simulink library "SimscapeCustomComponents_lib"  (R2025b)
settings: Solver=VariableStepAuto  StartTime=0.0  StopTime=10.0  RelTol=1e-3
undefined symbols (not defined in the file or in its folder): base, baseVdc, capacity, DiscIntNeverNeededParam, ee_sli_rtmsupport, filterInductance, freqeuncy, frequency, gcbh, gflInverter, gfmInverter, iMaxPU, Inertia, initialSOC, plantRating, solar, Ts, ups, Vac, windSystem, windTurbine
libraries: fl_lib x397, nesl_utility x171, eeGeneralControl x85, ee_lib x82, simulink x72, datacenter_lib x68, eeTransforms x38, slpidlib x24, buildingEnergy_lib x20, SimscapeFluids_lib x17, eeSinusoidalMeasurementV2 x8, eePwmGenerator x8
(part 4 of 24)

== system SimscapeCustomComponents_lib/Building Energy Management/Building/Room, Radiator, and Under-floor Piping ==
  Array Connection3 : SimscapeArrayConnection  Domain=foundation.thermal.thermal  NumScalarElements=6
  PS Selector : fl_lib/Physical Signals/Nonlinear Operators/PS Selector  ix=indxS
      settings: InternalSimscapePortConfiguration="{\"Bottom\":[],\"Left\":[{\"id\":\"I\",\"label\":\"\",\"type\":\"input\"}],\"Right\":[{\"id\":\"O\",\"label\":\"\",\"type\":\"output\"}],\"Top\":[]}"
  PS Selector1 : fl_lib/Physical Signals/Nonlinear Operators/PS Selector  ix=indxV
      settings: InternalSimscapePortConfiguration="{\"Bottom\":[],\"Left\":[{\"id\":\"I\",\"label\":\"\",\"type\":\"input\"}],\"Right\":[{\"id\":\"O\",\"label\":\"\",\"type\":\"output\"}],\"Top\":[]}"
  Room Underfloor Piping : buildingEnergy_lib/Room Underfloor Piping  pipeHydrDia=pipeHydrDiaUFP m  pipeLength=pipeLenUFP m  pipeArea=pipeCrossSectionalAreaUFP m^2  pipeRoughness=pipeRoughnessUFP m  htc=htc W/(K*m^2)  iniTemperature=iniT K
      settings: InternalSimscapePortConfiguration="{\"Bottom\":[],\"Left\":[{\"id\":\"TL_V\",\"label\":\"V\",\"type\":\"input\"},{\"id\":\"TL_A\",\"label\":\"A\",\"type\":\"foundation.thermal_liquid.thermal_liquid\"}],\"Right\":[{\"id\":\"M\",\"label\":\"R\",\"type\":\"foundation.thermal.thermal\"},{\"id\":\"TL_B\",\"label\":\"B\",\"type\":\"foundation.thermal_liquid.thermal_liquid\"}],\"Top\":[]}"
  Room Volume1 : buildingEnergy_lib/Room Volume  N1=1  N2=6  iniT=iniT K  length=roomLen m  width=roomWid m  height=roomHgt m
      settings: InternalSimscapePortConfiguration="{\"Bottom\":[],\"Left\":[{\"id\":\"S\",\"label\":\"S\",\"type\":\"input\"}],\"Right\":[{\"id\":\"T\",\"label\":\"T\",\"type\":\"output\"}],\"Top\":[{\"id\":\"M1\",\"label\":\"M1\",\"type\":\"foundation.thermal.thermal\"},{\"id\":\"M2\",\"label\":\"M2\",\"type\":\"foundation.thermal.thermal\"}]}"
  Room Wall Radiator : buildingEnergy_lib/Room Wall Radiator  pipeHydrDia=pipeHydrDiaR m  pipeLength=pipeLenR m  pipeArea=pipeCrossSectionalAreaR m^2  pipeRoughness=pipeRoughnessR m  htc=htc W/(K*m^2)  iniTemperature=iniT K
      settings: InternalSimscapePortConfiguration="{\"Bottom\":[],\"Left\":[{\"id\":\"TL_V\",\"label\":\"V\",\"type\":\"input\"},{\"id\":\"TL_A\",\"label\":\"A\",\"type\":\"foundation.thermal_liquid.thermal_liquid\"}],\"Right\":[{\"id\":\"M\",\"label\":\"R\",\"type\":\"foundation.thermal.thermal\"},{\"id\":\"TL_B\",\"label\":\"B\",\"type\":\"foundation.thermal_liquid.thermal_liquid\"}],\"Top\":[]}"
  Thermal Resistance : fl_lib/Thermal/Thermal Elements/Thermal Resistance  resistance=thermalResFloor K/W  T_specify=off  T_priority=None  T=0 K  T_nominal_specify=off  T_nominal_value=1  T_nominal_unit=K  Q_specify=off  Q_priority=None  Q=0 W  Q_nominal_specify=off  Q_nominal_value=1  Q_nominal_unit=W
  ar1 : fl_lib/Thermal/Thermal Elements/Convective Heat Transfer  thermal_type=foundation.enum.constant_variable.constant  area=roomLen*roomWid m^2  heat_tr_coeff=htc W/(K*m^2)  min_heat_tr_coeff=1e-3 W/(K*m^2)  T_specify=off  T_priority=None  T=0 K  T_nominal_specify=off  T_nominal_value=1  T_nominal_unit=K  Q_specify=off  Q_priority=None  Q=0 W  Q_nominal_specify=off  Q_nominal_value=1  Q_nominal_unit=W
  ar3 : fl_lib/Thermal/Thermal Elements/Convective Heat Transfer  thermal_type=foundation.enum.constant_variable.constant  area=roomHgt*roomWid m^2  heat_tr_coeff=htc W/(K*m^2)  min_heat_tr_coeff=1e-3 W/(K*m^2)  T_specify=off  T_priority=None  T=0 K  T_nominal_specify=off  T_nominal_value=1  T_nominal_unit=K  Q_specify=off  Q_priority=None  Q=0 W  Q_nominal_specify=off  Q_nominal_value=1  Q_nominal_unit=W
  ar4 : fl_lib/Thermal/Thermal Elements/Convective Heat Transfer  thermal_type=foundation.enum.constant_variable.constant  area=roomLen*roomHgt m^2  heat_tr_coeff=htc W/(K*m^2)  min_heat_tr_coeff=1e-3 W/(K*m^2)  T_specify=off  T_priority=None  T=0 K  T_nominal_specify=off  T_nominal_value=1  T_nominal_unit=K  Q_specify=off  Q_priority=None  Q=0 W  Q_nominal_specify=off  Q_nominal_value=1  Q_nominal_unit=W
  ar5 : fl_lib/Thermal/Thermal Elements/Convective Heat Transfer  thermal_type=foundation.enum.constant_variable.constant  area=roomHgt*roomWid m^2  heat_tr_coeff=htc W/(K*m^2)  min_heat_tr_coeff=1e-3 W/(K*m^2)  T_specify=off  T_priority=None  T=0 K  T_nominal_specify=off  T_nominal_value=1  T_nominal_unit=K  Q_specify=off  Q_priority=None  Q=0 W  Q_nominal_specify=off  Q_nominal_value=1  Q_nominal_unit=W
  ar6 : fl_lib/Thermal/Thermal Elements/Convective Heat Transfer  thermal_type=foundation.enum.constant_variable.constant  area=roomLen*roomHgt m^2  heat_tr_coeff=htc W/(K*m^2)  min_heat_tr_coeff=1e-3 W/(K*m^2)  T_specify=off  T_priority=None  T=0 K  T_nominal_specify=off  T_nominal_value=1  T_nominal_unit=K  Q_specify=off  Q_priority=None  Q=0 W  Q_nominal_specify=off  Q_nominal_value=1  Q_nominal_unit=W
  ar7 : fl_lib/Thermal/Thermal Elements/Convective Heat Transfer  thermal_type=foundation.enum.constant_variable.constant  area=pipeLenR*pipeHydrDiaR m^2  heat_tr_coeff=htc W/(K*m^2)  min_heat_tr_coeff=1e-3 W/(K*m^2)  T_specify=off  T_priority=None  T=0 K  T_nominal_specify=off  T_nominal_value=1  T_nominal_unit=K  Q_specify=off  Q_priority=None  Q=0 W  Q_nominal_specify=off  Q_nominal_value=1  Q_nominal_unit=W
  ar8 : fl_lib/Thermal/Thermal Elements/Convective Heat Transfer  thermal_type=foundation.enum.constant_variable.constant  area=pipeLenUFP*pipeHydrDiaUFP/2 m^2  heat_tr_coeff=htc W/(K*m^2)  min_heat_tr_coeff=1e-3 W/(K*m^2)  T_specify=off  T_priority=None  T=0 K  T_nominal_specify=off  T_nominal_value=1  T_nominal_unit=K  Q_specify=off  Q_priority=None  Q=0 W  Q_nominal_specify=off  Q_nominal_value=1  Q_nominal_unit=W
  V : PMIOPort  Side=Left
  S : PMIOPort  Port=2  Side=Left
  W4 : PMIOPort  Port=3  Side=Left
  TL_A : PMIOPort  Port=4  Side=Left
  W3 : PMIOPort  Port=5  Side=Left
  TL_B : PMIOPort  Port=6  Side=Right
  W2 : PMIOPort  Port=7  Side=Right
  T : PMIOPort  Port=8  Side=Right
  W1 : PMIOPort  Port=9  Side=Right
  Bottom : PMIOPort  Port=10  Side=Right
  Top : PMIOPort  Port=11  Side=Left
  connections:
  TL_B/RConn1 -- Room Underfloor Piping/RConn2 -- Room Wall Radiator/RConn2
  Room Volume1/RConn1 -- T/RConn1
  TL_A/RConn1 -- Room Underfloor Piping/LConn2 -- Room Wall Radiator/LConn2
  ar6/RConn1 -- W1/RConn1
  ar5/RConn1 -- W2/RConn1
  ar4/RConn1 -- W3/RConn1
  ar3/RConn1 -- W4/RConn1
  Thermal Resistance/LConn1 -- Room Underfloor Piping/RConn1 -- ar8/LConn1
  ar7/RConn1 -- Array Connection3/LConn2
  Top/RConn1 -- ar1/RConn1
  Thermal Resistance/RConn1 -- Bottom/RConn1
  Array Connection3/LConn3 -- ar3/LConn1
  Array Connection3/LConn4 -- ar4/LConn1
  Array Connection3/LConn5 -- ar5/LConn1
  Array Connection3/LConn6 -- ar6/LConn1
  Room Wall Radiator/RConn1 -- ar7/LConn1
  ar8/RConn1 -- Array Connection3/LConn1
  V/RConn1 -- PS Selector1/LConn1
  PS Selector1/RConn1 -- Room Underfloor Piping/LConn1 -- Room Wall Radiator/LConn1
  Room Volume1/LConn1 -- PS Selector/RConn1
  PS Selector/LConn1 -- S/RConn1
  Room Volume1/LConn3 -- Array Connection3/RConn1
  ar1/LConn1 -- Room Volume1/LConn2

== system SimscapeCustomComponents_lib/Building Energy Management/HVAC/Air Water Heat Pump (TL) ==
  ActualFlowrate : fl_lib/Physical Signals/Nonlinear Operators/PS Max  ZeroCross=true
      settings: InternalSimscapePortConfiguration="{\"Bottom\":[],\"Left\":[{\"id\":\"I1\",\"label\":\"\",\"type\":\"input\"},{\"id\":\"I2\",\"label\":\"\",\"type\":\"input\"}],\"Right\":[{\"id\":\"O\",\"label\":\"\",\"type\":\"output\"}],\"Top\":[]}"
  Air Water Heat Pump : buildingEnergy_lib/Air Water Heat Pump  nominalCapacityA=heatingCapacityA kW  seasonalCOPvalA=heatingCoPA  nominalCapacityB=heatingCapacityB kW  seasonalCOPvalB=heatingCoPB  nominalCapacityC=heatingCapacityC kW  seasonalCOPvalC=heatingCoPC  nominalCapacityD=heatingCapacityD kW  seasonalCOPvalD=heatingCoPD  nominalCapacityE=coolingCapacityE kW  seasonalCOPvalE=coolingCoPE  nominalCapacityF=coolingCapacityF kW  seasonalCOPvalF=coolingCoPF  backupElecHeater=elecHeaterPower kW  wInletOpRangeUpp=waterOpTempMax K  wInletOpRangeLow=waterOpTempMin K  airTemperatureVector=273 + [-2, -2, 7, 7, 35, 35]  waterTemperatureVector=273 + [55, 65, 35, 45, 18, 7]  waterSpHeat=4186 J/(K*kg)  smallPower=1e-3 W  maxCOP_specify=off  maxCOP_priority=None  maxCOP=8  maxCOP_nominal_specify=off  maxCOP_nominal_value=1  maxCOP_nominal_unit=1
      settings: InternalSimscapePortConfiguration="{\"Bottom\":[{\"id\":\"Ta\",\"label\":\"Ta\",\"type\":\"input\"},{\"id\":\"Tw\",\"label\":\"Tw\",\"type\":\"input\"}],\"Left\":[{\"id\":\"Tl\",\"label\":\"Tl\",\"type\":\"input\"},{\"id\":\"Fw\",\"label\":\"Fw\",\"type\":\"input\"},{\"id\":\"Op\",\"label\":\"Op\",\"type\":\"input\"},{\"id\":\"Ep\",\"label\":\"Ep\",\"type\":\"input\"},{\"id\":\"Nd\",\"label\":\"Nd\",\"type\":\"input\"}],\"Right\":[{\"id\":\"calcCap\",\"label\":\"Q\",\"type\":\"output\"},{\"id\":\"calcCOP\",\"label\":\"COP\",\"type\":\"output\"},{\"id\":\"ePower\",\"label\":\"ePow\",\"type\":\"output\"}],\"Top\":[]}"
  Heat : fl_lib/Thermal/Thermal Sources/Controlled Heat Flow Rate Source
  InMeasDelay : fl_lib/Physical Signals/Linear Operators/PS Transfer Function  transfer_function_type=foundation.enum.transfer_function_type.lag  T=measTimelagWater s  T1=2 s  T2=1 s  reset_method=foundation.enum.IntegratorResetSpec.None  initial_condition_spec=foundation.enum.IntegratorICSpec.Internal  y0=initialT K
      settings: InternalSimscapePortConfiguration="{\"Bottom\":[],\"Left\":[{\"id\":\"U\",\"label\":\"\",\"type\":\"input\"}],\"Right\":[{\"id\":\"Y\",\"label\":\"\",\"type\":\"output\"}],\"Top\":[]}"
  InsTank : fl_lib/Thermal/Thermal Elements/Perfect Insulator  T_specify=off  T_priority=None  T=293.15 K  T_nominal_specify=off  T_nominal_value=1  T_nominal_unit=K
  InternalCoils : fl_lib/Thermal Liquid/Elements/Pipe (TL)  length=coilLen m  area=coilArea m^2  Dh=coilDia m  length_add=0 m  roughness=15e-6 m  Re_lam=2000  Re_tur=4000  shape_factor=64  Nu_lam=3.66  dynamic_compressibility=true  inertia=false  p0=initialP MPa  T0=initialT K  mdot0=0 kg/s  p_nominal=0.101325 MPa  T_nominal=293.15 K
  MinFlowValue : fl_lib/Physical Signals/Sources/PS Constant  constant=minWaterFlowRate kg/s
  NoDeviation : fl_lib/Physical Signals/Sources/PS Constant  constant=1
  NomDevLim : fl_lib/Physical Signals/Nonlinear Operators/PS Max  ZeroCross=true
      settings: InternalSimscapePortConfiguration="{\"Bottom\":[],\"Left\":[{\"id\":\"I1\",\"label\":\"\",\"type\":\"input\"},{\"id\":\"I2\",\"label\":\"\",\"type\":\"input\"}],\"Right\":[{\"id\":\"O\",\"label\":\"\",\"type\":\"output\"}],\"Top\":[]}"
  OutMeasDelay : fl_lib/Physical Signals/Linear Operators/PS Transfer Function  transfer_function_type=foundation.enum.transfer_function_type.lag  T=measTimelagWater s  T1=2 s  T2=1 s  reset_method=foundation.enum.IntegratorResetSpec.None  initial_condition_spec=foundation.enum.IntegratorICSpec.Internal  y0=initialT K
      settings: InternalSimscapePortConfiguration="{\"Bottom\":[],\"Left\":[{\"id\":\"U\",\"label\":\"\",\"type\":\"input\"}],\"Right\":[{\"id\":\"Y\",\"label\":\"\",\"type\":\"output\"}],\"Top\":[]}"
  Tank : SimscapeFluids_lib/Thermal Liquid/Tanks & Accumulators/Gas-Charged Accumulator (TL)  capacity=tankVolume m^3  dead_volume=4e-5 m^3  p_precharge_gauge=0 MPa  k_sh=1.4  area=0.01 m^2  stiff_coeff=1e4 MPa/m^3  damping_coeff=1e4 MPa*s/m^6  liquid_volume_specify=off  liquid_volume_priority=High  liquid_volume=5e-3 m^3  liquid_volume_nominal_specify=off  liquid_volume_nominal_value=1  liquid_volume_nominal_unit=m^3  liquid_mass_specify=off  liquid_mass_priority=None  liquid_mass=5 kg  liquid_mass_nominal_specify=off  liquid_mass_nominal_value=1  liquid_mass_nominal_unit=kg  p_I_specify=off  p_I_priority=None  p_I=0.101325 MPa  p_I_nominal_specify=off  p_I_nominal_value=1  p_I_nominal_unit=MPa  T_I_specify=on  T_I_priority=High  T_I=initialT K  T_I_nominal_specify=off  T_I_nominal_value=1  T_I_nominal_unit=K
      settings: InternalSimscapePortConfiguration="{\"Bottom\":[],\"Left\":[],\"Right\":[{\"id\":\"A\",\"label\":\"A\",\"type\":\"foundation.thermal_liquid.thermal_liquid\"},{\"id\":\"H\",\"label\":\"H\",\"type\":\"foundation.thermal.thermal\"}],\"Top\":[]}"
  Tref : fl_lib/Thermal/Thermal Elements/Thermal Reference
  TwInet : fl_lib/Thermal Liquid/Sensors/Pressure & Temperature Sensor (TL)  reference=foundation.enum.MeasurementReference.absolute  pressure=false  pressure_spec=foundation.enum.PressureMeasementSpec.Absolute  temperature=true
      settings: InternalSimscapePortConfiguration="{\"Bottom\":[{\"id\":\"T\",\"label\":\"T\",\"type\":\"output\"}],\"Left\":[{\"id\":\"A\",\"label\":\"A\",\"type\":\"foundation.thermal_liquid.thermal_liquid\"}],\"Right\":[],\"Top\":[]}"
  TwOut : fl_lib/Thermal Liquid/Sensors/Pressure & Temperature Sensor (TL)  reference=foundation.enum.MeasurementReference.absolute  pressure=false  pressure_spec=foundation.enum.PressureMeasementSpec.Absolute  temperature=true
      settings: InternalSimscapePortConfiguration="{\"Bottom\":[{\"id\":\"T\",\"label\":\"T\",\"type\":\"output\"}],\"Left\":[{\"id\":\"A\",\"label\":\"A\",\"type\":\"foundation.thermal_liquid.thermal_liquid\"}],\"Right\":[],\"Top\":[]}"
  WaterFlowRate : fl_lib/Thermal Liquid/Sources/Flow Rate Source (TL)  source_type=foundation.enum.constant_controlled.controlled  flow_type=foundation.enum.mass_volumetric_flow.mass  mass_flow=0 kg/s  volumetric_flow=0 m^3/s  power_spec=foundation.enum.power_spec.none  area=coilArea m^2
  Fw : PMIOPort  Side=Left
  Ta : PMIOPort  Port=2  Side=Left
  Op : PMIOPort  Port=3  Side=Left
  Ep : PMIOPort  Port=4  Side=Left
  Nd : PMIOPort  Port=5  Side=Left
  A : PMIOPort  Port=6  Side=Right
  B : PMIOPort  Port=7  Side=Right
  ePow : PMIOPort  Port=8  Side=Right
  COP : PMIOPort  Port=9  Side=Right
  connections:
  TwOut/LConn1 -- B/RConn1 -- InternalCoils/RConn1
  InternalCoils/LConn1 -- WaterFlowRate/RConn1 -- TwInet/LConn1
  Fw/RConn1 -- Air Water Heat Pump/LConn2 -- ActualFlowrate/LConn1
  WaterFlowRate/LConn1 -- A/RConn1 -- Tank/RConn1
  Air Water Heat Pump/LConn1 -- InMeasDelay/RConn1
  Air Water Heat Pump/LConn3 -- Op/RConn1
  InMeasDelay/LConn1 -- TwInet/RConn1
  InternalCoils/LConn2 -- Heat/RConn2
  ePow/RConn1 -- Air Water Heat Pump/RConn3
  InsTank/LConn1 -- Tank/RConn2
  NoDeviation/RConn1 -- NomDevLim/LConn2
  Air Water Heat Pump/LConn4 -- Ep/RConn1
  Air Water Heat Pump/RConn2 -- COP/RConn1
  ActualFlowrate/RConn1 -- WaterFlowRate/LConn2
  MinFlowValue/RConn1 -- ActualFlowrate/LConn2
  Air Water Heat Pump/RConn5 -- OutMeasDelay/RConn1
  Tref/LConn1 -- Heat/LConn1
  Air Water Heat Pump/LConn5 -- NomDevLim/RConn1
  TwOut/RConn1 -- OutMeasDelay/LConn1
  Nd/RConn1 -- NomDevLim/LConn1
  Air Water Heat Pump/RConn4 -- Ta/RConn1
  Heat/RConn1 -- Air Water Heat Pump/RConn1

== system SimscapeCustomComponents_lib/Building Energy Management/HVAC/Heat Source Control ==
  HeatPumpCapacity : fl_lib/Physical Signals/Sources/PS Constant  constant=capacity J/s
  MeasurementDelay : fl_lib/Physical Signals/Linear Operators/PS Transfer Function  transfer_function_type=foundation.enum.transfer_function_type.lag  T=tau s  T1=2 s  T2=1 s  reset_method=foundation.enum.IntegratorResetSpec.None  initial_condition_spec=foundation.enum.IntegratorICSpec.Internal  y0=iniT K
      settings: InternalSimscapePortConfiguration="{\"Bottom\":[],\"Left\":[{\"id\":\"U\",\"label\":\"\",\"type\":\"input\"}],\"Right\":[{\"id\":\"Y\",\"label\":\"\",\"type\":\"output\"}],\"Top\":[]}"
  NumHeatPump : fl_lib/Physical Signals/Functions/PS Gain  gain=num
  PS Divide : fl_lib/Physical Signals/Functions/PS Divide
  PS Product : fl_lib/Physical Signals/Functions/PS Product
  PS Subtract : fl_lib/Physical Signals/Functions/PS Subtract
  PS Sum of Elements : fl_lib/Physical Signals/Functions/PS Sum of Elements  sumAll=true
      settings: InternalSimscapePortConfiguration="{\"Bottom\":[],\"Left\":[{\"id\":\"I\",\"label\":\"\",\"type\":\"input\"}],\"Right\":[{\"id\":\"O\",\"label\":\"\",\"type\":\"output\"}],\"Top\":[]}"
  PS Sum of Elements2 : fl_lib/Physical Signals/Functions/PS Sum of Elements  sumAll=true
      settings: InternalSimscapePortConfiguration="{\"Bottom\":[],\"Left\":[{\"id\":\"I\",\"label\":\"\",\"type\":\"input\"}],\"Right\":[{\"id\":\"O\",\"label\":\"\",\"type\":\"output\"}],\"Top\":[]}"
  Values<0 : fl_lib/Physical Signals/Nonlinear Operators/PS Saturation  upper_limit=0 J/s  lower_limit=-inf J/s  ZeroCross=true
  Values>0 : fl_lib/Physical Signals/Nonlinear Operators/PS Saturation  upper_limit=inf J/s  lower_limit=0 J/s  ZeroCross=true
  WaterTchange : fl_lib/Physical Signals/Sources/PS Constant  constant=delT K
  Cooling : PMIOPort  Side=Left
  Heating : PMIOPort  Port=2  Side=Left
  S : PMIOPort  Port=3  Side=Left
  Ts : PMIOPort  Port=4  Side=Right
  Tr : PMIOPort  Port=5  Side=Right
  connections:
  PS Subtract/RConn1 -- PS Product/LConn1
  Tr/RConn1 -- MeasurementDelay/LConn1
  PS Subtract/LConn1 -- Ts/RConn1
  Heating/RConn1 -- PS Sum of Elements/RConn1
  Cooling/RConn1 -- PS Sum of Elements2/RConn1
  PS Sum of Elements/LConn1 -- Values>0/RConn1
  PS Sum of Elements2/LConn1 -- Values<0/RConn1
  MeasurementDelay/RConn1 -- PS Subtract/LConn2
  HeatPumpCapacity/RConn1 -- PS Divide/LConn1
  WaterTchange/RConn1 -- PS Divide/LConn2
  NumHeatPump/LConn1 -- PS Divide/RConn1
  NumHeatPump/RConn1 -- PS Product/LConn2
  S/RConn1 -- Values<0/LConn1 -- Values>0/LConn1 -- PS Product/RConn1

== system SimscapeCustomComponents_lib/Datacenter/Assemblies/Air Cooled PDU Assembly ==
  One : fl_lib/Physical Signals/Sources/PS Constant  constant=1
  PDU Racks : Subsystem  mask{nTrays=nTrays, nRacks=nRacks, trayMass=trayMass, trayCp=trayCp, trayThermalR=trayThermalR, nGPU=nGPU, gpuTDPperDie=gpuTDPperDie, gpuIdlePower=gpuIdlePower, gpuHBMpower=gpuHBMpower, gpuExponent=gpuExponent, gpuHBMutil=gpuHBMutil, gpuLeakage=gpuLeakage, gpuNominalDieT=gpuNominalDieT, gpuDieThermalC=gpuDieThermalC, gpuHeatSinkR=gpuHeatSinkR, gpuSurfArea=gpuSurfArea, gpuAmbientR=gpuAmbientR, nCPU=nCPU, cpuTDPperSocket=cpuTDPperSocket, cpuIdlePower=cpuIdlePower, cpuExponent=cpuExponent, cpuLeakage=cpuLeakage, cpuNominalDieT=cpuNominalDieT, cpuDieThermalC=cpuDieThermalC, cpuHeatSinkR=cpuHeatSinkR, cpuSurfArea=cpuSurfArea, cpuAmbientR=cpuAmbientR, initialT=initialT, htc=htc}
      mask prompts: nTrays "Number of IT trays per rack (-)"; nRacks "Number of racks (-)"; trayMass "Tray mass (kg)"; trayCp "Tray specific heat capacity (J/kg*K)"; trayThermalR "Tray to external thermal resistance (K/W)"; nGPU "Number of GPU per tray (-)"; gpuTDPperDie "GPU TDP per die (W)"; gpuIdlePower "GPU idle power (W)"; gpuHBMpower "HBM power per GPU (W)"; gpuExponent "GPU power utilization exponent (-)"; gpuHBMutil "HBM utilization as fraction of compute utilization (-)"; gpuLeakage "Leakage increase per K above nominal temperature (W/K)"; gpuNominalDieT "Nominal die temperature at TDP (K)"; gpuDieThermalC "GPU die thermal capacitance (J/K)"; gpuHeatSinkR "GPU die-heat-sink thermal resistance (K/W)"; gpuSurfArea "Surface area per die for ambient heat transfer (m^2)"; gpuAmbientR "GPU die-ambient thermal resistance (K/W)"; nCPU "Number of CPU per tray (-)"; cpuTDPperSocket "CPU TDP per socket (W)"; cpuIdlePower "CPU idle power per socket (W)"; cpuExponent "CPU power utilization exponent (-)"; cpuLeakage "Leakage increase per K above nominal temperature (W/K)"; cpuNominalDieT "Nominal die temperature at TDP (K)"; cpuDieThermalC "CPU die thermal capacitance (J/K)"; cpuHeatSinkR "CPU die-heat-sink thermal resistance (K/W)"; cpuSurfArea "Surface area per die for ambient heat transfer (m^2)"; cpuAmbientR "CPU die-ambient thermal resistance (K/W)"; initialT "Initial temperature (K)"; htc "Heat transfer coefficient to ambient (W/m^2.K)"
      settings: CopyFcn=set_param(gcbh,'LinkStatus','none');  PortSchema="{\"entries\":[{\"content\":{\"sides\":[{\"content\":{\"connectorIds\":[\"LConn1\",\"LConn2\",\"LConn3\"]},\"type\":\"ConnectorPlacement.EquallySpacedRectSide\",\"uuid\":\"1a9a884a-dab1-4495-bf62-c6b2de6c1039\"},{\"content\":{\"connectorIds\":[\"RConn1\",\"RConn2\",\"RConn3\"],\"side\":\"RIGHT\"},\"type\":\"ConnectorPlacement.EquallySpacedRectSide\",\"uuid\":\"05c53434-51c1-4fee-b885-c321dcda8b6b\"},{\"content\":{\"side\":\"TOP\"},\"type\":\"ConnectorPlacement.EquallySpacedRectSide\",\"uuid\":\"c7b5c534-d596-4858-a133-27f005e6c9d4\"},{\"content\":{\"connectorIds\":[\"RConn4\"],\"side\":\"BOTTOM\"},\"type\":\"ConnectorPlacement.EquallySpacedRectSide\",\"uuid\":\"693f3c99-4296-4d86-bfcc-da753d3e576f\"}]},\"type\":\"ConnectorPlacement.EquallySpacedConnector\",\"uuid\":\"ed91c467-c4d0-403f-af16-bac0257594fd\"}],\"packageUris\":[\"http://schema.mathworks.com/mf0/Connector/R2020b\"],\"version\":\"1.0\"}"
      mask Help: web("DocumentationPDURacks.html")
      mask DialogControl Container10 Prompt: PDU Racks
      mask DialogControl getRatingButton Prompt: Get Rating
      mask DialogControl Container9 Prompt: IT Tray
      mask DialogControl Container6 Prompt: GPU
      mask DialogControl Container7 Prompt: CPU
      mask DialogControl Container8 Prompt: Initial Conditions
      mask Display: image('icon_PDURacks.png');
  PS Product1 : fl_lib/Physical Signals/Functions/PS Product
  PS Product2 : fl_lib/Physical Signals/Functions/PS Product
  Rack Air Cooling : Subsystem  mask{nFans=nFans, flowVec=flowVec, prDropVec=prDropVec, fanEffVec=fanEffVec, fluidDen=1.28, fluidCp=1005}
      mask prompts: nFans "Number of fans (-)"; flowVec "Fan flow rate vector (m^3/s)"; prDropVec "Pressure drop vector (Pa)"; fanEffVec "Fan efficiency vector (-)"; fluidDen "Fluid density (kg/m^3)"; fluidCp "Fluid heat capacity (J/(Kg*K))"
      settings: CopyFcn=set_param(gcbh,'LinkStatus','none');
      mask Help: web("DocumentationRackAirCooling.html")
      mask DialogControl Container3 Prompt: Fans
      mask DialogControl Container4 Prompt: Fluid Properties
      mask Display: image('icon_PDUfanCooling.png');
  Thermal Multiplier : datacenter_lib/Thermal Multiplier
      settings: InternalSimscapePortConfiguration="{\"Bottom\":[],\"Left\":[{\"id\":\"A\",\"label\":\"A\",\"type\":\"foundation.thermal.thermal\"}],\"Right\":[{\"id\":\"B\",\"label\":\"B\",\"type\":\"foundation.thermal.thermal\"}],\"Top\":[{\"id\":\"Na\",\"label\":\"Na\",\"type\":\"input\"},{\"id\":\"Nb\",\"label\":\"Nb\",\"type\":\"input\"}]}"
  Thermal Multiplier1 : datacenter_lib/Thermal Multiplier
      settings: InternalSimscapePortConfiguration="{\"Bottom\":[],\"Left\":[{\"id\":\"A\",\"label\":\"A\",\"type\":\"foundation.thermal.thermal\"}],\"Right\":[{\"id\":\"B\",\"label\":\"B\",\"type\":\"foundation.thermal.thermal\"}],\"Top\":[{\"id\":\"Na\",\"label\":\"Na\",\"type\":\"input\"},{\"id\":\"Nb\",\"label\":\"Nb\",\"type\":\"input\"}]}"
  nAssemblies : fl_lib/Physical Signals/Sources/PS Constant  constant=nAssembly
  U_gpu : PMIOPort  Side=Left
  U_cpu : PMIOPort  Port=2  Side=Left
  S_fan : PMIOPort  Port=3  Side=Left
  T_gpu : PMIOPort  Port=4  Side=Right
  T_cpu : PMIOPort  Port=5  Side=Right
  P_pdu : PMIOPort  Port=6  Side=Right
  P_fan : PMIOPort  Port=7  Side=Right
  C : PMIOPort  Port=8  Side=Left
  H : PMIOPort  Port=9  Side=Right
  connections:
  Rack Air Cooling/RConn1 -- PDU Racks/RConn4
  PDU Racks/RConn3 -- T_cpu/RConn1
  PDU Racks/LConn2 -- U_cpu/RConn1
  PDU Racks/RConn2 -- T_gpu/RConn1
  Rack Air Cooling/LConn2 -- S_fan/RConn1
  PDU Racks/LConn1 -- U_gpu/RConn1
  Thermal Multiplier/RConn1 -- PDU Racks/LConn3
  nAssemblies/RConn1 -- Thermal Multiplier1/LConn3 -- PS Product1/LConn1 -- PS Product2/LConn1 -- Thermal Multiplier/LConn3
  One/RConn1 -- Thermal Multiplier1/LConn2 -- Thermal Multiplier/LConn2
  P_pdu/RConn1 -- PS Product1/RConn1
  PS Product1/LConn2 -- PDU Racks/RConn1
  PS Product2/RConn1 -- P_fan/RConn1
  PS Product2/LConn2 -- Rack Air Cooling/RConn2
  Thermal Multiplier1/RConn1 -- Rack Air Cooling/LConn1
  H/RConn1 -- Thermal Multiplier/LConn1
  C/RConn1 -- Thermal Multiplier1/LConn1

== system SimscapeCustomComponents_lib/Datacenter/Assemblies/PDU + CDU Assembly (LUT) ==
  CDU (LUT) : Subsystem  mask{numPump=numPump, flowrate_vec=flowrate_vec, capacity_vec=capacity_vec, effPump_vec=effPump_vec, prDrop_mat=prDrop_mat, speed=speed}
      mask prompts: numPump "Total number of pumps (-)"; flowrate_vec "Coolant volumetric flowrate vector (m^3/s)"; capacity_vec "Heat exchanger capacity vector (W)"; effPump_vec "Pump efficiency vector, 0-1 (-)"; prDrop_mat "Pressure drop (Pa)"; speed "Pump speed scaling (-)"
      settings: CopyFcn=set_param(gcbh,'LinkStatus','none');  PortSchema="{\"entries\":[{\"content\":{\"sides\":[{\"content\":{\"connectorIds\":[\"LConn1\",\"LConn2\"]},\"type\":\"ConnectorPlacement.EquallySpacedRectSide\",\"uuid\":\"dd9276e8-a048-49df-a05c-f18b45aafce3\"},{\"content\":{\"connectorIds\":[\"RConn1\",\"RConn2\"],\"side\":\"RIGHT\"},\"type\":\"ConnectorPlacement.EquallySpacedRectSide\",\"uuid\":\"f4cbe01b-cfd4-4d60-aff7-a07955033ed5\"},{\"content\":{\"connectorIds\":[\"LConn3\"],\"side\":\"TOP\"},\"type\":\"ConnectorPlacement.EquallySpacedRectSide\",\"uuid\":\"ad27df56-4241-452c-8570-6a66062dd2f2\"}]},\"type\":\"ConnectorPlacement.EquallySpacedConnector\",\"uuid\":\"0333b5f9-1896-45e0-922d-790b0e5dd980\"}],\"packageUris\":[\"http://schema.mathworks.com/mf0/Connector/R2020b\"],\"version\":\"1.0\"}"
      mask Help: web("DocumentationCDULUT.html")
      mask DialogControl Container4 Prompt: CDU
      mask Display: image('icon_CDUtableBased.png');
  One : fl_lib/Physical Signals/Sources/PS Constant  constant=1
  PDU Racks : Subsystem  mask{nTrays=nTrays, nRacks=nRacks, trayMass=trayMass, trayCp=trayCp, trayThermalR=trayThermalR, nGPU=nGPU, gpuTDPperDie=gpuTDPperDie, gpuIdlePower=gpuIdlePower, gpuHBMpower=gpuHBMpower, gpuExponent=gpuExponent, gpuHBMutil=gpuHBMutil, gpuLeakage=gpuLeakage, gpuNominalDieT=gpuNominalDieT, gpuDieThermalC=gpuDieThermalC, gpuHeatSinkR=gpuHeatSinkR, gpuSurfArea=gpuSurfArea, gpuAmbientR=gpuAmbientR, nCPU=nCPU, cpuTDPperSocket=cpuTDPperSocket, cpuIdlePower=cpuIdlePower, cpuExponent=cpuExponent, cpuLeakage=cpuLeakage, cpuNominalDieT=cpuNominalDieT, cpuDieThermalC=cpuDieThermalC, cpuHeatSinkR=cpuHeatSinkR, cpuSurfArea=cpuSurfArea, cpuAmbientR=cpuAmbientR, initialT=initialT, htc=htc}
      mask prompts: nTrays "Number of IT trays per rack (-)"; nRacks "Number of racks (-)"; trayMass "Tray mass (kg)"; trayCp "Tray specific heat capacity (J/kg*K)"; trayThermalR "Tray to external thermal resistance (K/W)"; nGPU "Number of GPU per tray (-)"; gpuTDPperDie "GPU TDP per die (W)"; gpuIdlePower "GPU idle power (W)"; gpuHBMpower "HBM power per GPU (W)"; gpuExponent "GPU power utilization exponent (-)"; gpuHBMutil "HBM utilization as fraction of compute utilization (-)"; gpuLeakage "Leakage increase per K above nominal temperature (W/K)"; gpuNominalDieT "Nominal die temperature at TDP (K)"; gpuDieThermalC "GPU die thermal capacitance (J/K)"; gpuHeatSinkR "GPU die-heat-sink thermal resistance (K/W)"; gpuSurfArea "Surface area per die for ambient heat transfer (m^2)"; gpuAmbientR "GPU die-ambient thermal resistance (K/W)"; nCPU "Number of CPU per tray (-)"; cpuTDPperSocket "CPU TDP per socket (W)"; cpuIdlePower "CPU idle power per socket (W)"; cpuExponent "CPU power utilization exponent (-)"; cpuLeakage "Leakage increase per K above nominal temperature (W/K)"; cpuNominalDieT "Nominal die temperature at TDP (K)"; cpuDieThermalC "CPU die thermal capacitance (J/K)"; cpuHeatSinkR "CPU die-heat-sink thermal resistance (K/W)"; cpuSurfArea "Surface area per die for ambient heat transfer (m^2)"; cpuAmbientR "CPU die-ambient thermal resistance (K/W)"; initialT "Initial temperature (K)"; htc "Heat transfer coefficient to ambient (W/m^2.K)"
      settings: CopyFcn=set_param(gcbh,'LinkStatus','none');  PortSchema="{\"entries\":[{\"content\":{\"sides\":[{\"content\":{\"connectorIds\":[\"LConn1\",\"LConn2\",\"LConn3\"]},\"type\":\"ConnectorPlacement.EquallySpacedRectSide\",\"uuid\":\"1a9a884a-dab1-4495-bf62-c6b2de6c1039\"},{\"content\":{\"connectorIds\":[\"RConn1\",\"RConn2\",\"RConn3\"],\"side\":\"RIGHT\"},\"type\":\"ConnectorPlacement.EquallySpacedRectSide\",\"uuid\":\"05c53434-51c1-4fee-b885-c321dcda8b6b\"},{\"content\":{\"side\":\"TOP\"},\"type\":\"ConnectorPlacement.EquallySpacedRectSide\",\"uuid\":\"c7b5c534-d596-4858-a133-27f005e6c9d4\"},{\"content\":{\"connectorIds\":[\"RConn4\"],\"side\":\"BOTTOM\"},\"type\":\"ConnectorPlacement.EquallySpacedRectSide\",\"uuid\":\"693f3c99-4296-4d86-bfcc-da753d3e576f\"}]},\"type\":\"ConnectorPlacement.EquallySpacedConnector\",\"uuid\":\"ed91c467-c4d0-403f-af16-bac0257594fd\"}],\"packageUris\":[\"http://schema.mathworks.com/mf0/Connector/R2020b\"],\"version\":\"1.0\"}"
      mask Help: web("DocumentationPDURacks.html")
      mask DialogControl Container10 Prompt: PDU Racks
      mask DialogControl getRatingButton Prompt: Get Rating
      mask DialogControl Container9 Prompt: IT Tray
      mask DialogControl Container6 Prompt: GPU
      mask DialogControl Container7 Prompt: CPU
      mask DialogControl Container8 Prompt: Initial Conditions
      mask Display: image('icon_PDURacks.png');
  PS Product : fl_lib/Physical Signals/Functions/PS Product
  PS Product1 : fl_lib/Physical Signals/Functions/PS Product
  PS Product2 : fl_lib/Physical Signals/Functions/PS Product
  Thermal Multiplier : datacenter_lib/Thermal Multiplier
      settings: InternalSimscapePortConfiguration="{\"Bottom\":[],\"Left\":[{\"id\":\"A\",\"label\":\"A\",\"type\":\"foundation.thermal.thermal\"}],\"Right\":[{\"id\":\"B\",\"label\":\"B\",\"type\":\"foundation.thermal.thermal\"}],\"Top\":[{\"id\":\"Na\",\"label\":\"Na\",\"type\":\"input\"},{\"id\":\"Nb\",\"label\":\"Nb\",\"type\":\"input\"}]}"
  nAssemblies : fl_lib/Physical Signals/Sources/PS Constant  constant=nAssembly
  U_gpu : PMIOPort  Side=Left
  U_cpu : PMIOPort  Port=2  Side=Left
  S_cdu : PMIOPort  Port=3  Side=Left
  N_cdu : PMIOPort  Port=4  Side=Left
  H : PMIOPort  Port=5  Side=Left
  T_gpu : PMIOPort  Port=6  Side=Right
  T_cpu : PMIOPort  Port=7  Side=Right
  P_pdu : PMIOPort  Port=8  Side=Right
  P_cdu : PMIOPort  Port=9  Side=Right
  Q_cdu : PMIOPort  Port=10  Side=Right
  connections:
  CDU (LUT)/LConn2 -- N_cdu/RConn1
  CDU (LUT)/LConn3 -- PDU Racks/RConn4
  PDU Racks/LConn1 -- U_gpu/RConn1
  CDU (LUT)/LConn1 -- S_cdu/RConn1
  PDU Racks/LConn2 -- U_cpu/RConn1
  Thermal Multiplier/LConn1 -- H/RConn1
  Thermal Multiplier/RConn1 -- PDU Racks/LConn3
  nAssemblies/RConn1 -- PS Product2/LConn1 -- PS Product1/LConn1 -- PS Product/LConn1 -- Thermal Multiplier/LConn3
  One/RConn1 -- Thermal Multiplier/LConn2
  PS Product/LConn2 -- PDU Racks/RConn1
  PS Product1/LConn2 -- CDU (LUT)/RConn1
  PS Product2/RConn1 -- Q_cdu/RConn1
  PS Product2/LConn2 -- CDU (LUT)/RConn2
  T_gpu/RConn1 -- PDU Racks/RConn2
  T_cpu/RConn1 -- PDU Racks/RConn3
  P_pdu/RConn1 -- PS Product/RConn1
  P_cdu/RConn1 -- PS Product1/RConn1

== system SimscapeCustomComponents_lib/Datacenter/Assemblies/PDU + CDU Assembly (TL) ==
  CDU (TL) : Subsystem  mask{extFluidMdot=extFluidMdot, extFluidPrDrop=extFluidPrDrop, extFluidVol=extFluidVol, extFluidPipeArea=extFluidPipeArea, intFluidMdot=intFluidMdot, intFluidPrDrop=intFluidPrDrop, intFluidVol=intFluidVol, intFluidPipeArea=intFluidPipeArea, spDissipationTbl=spDissipationTbl, effPipeLen=effPipeLen, pumpCapacityVec=pumpCapacityVec, pumpRefHeadVec=pumpRefHeadVec, pumpRefBrkPowVec=pumpRefBrkPowVec, pumpEff=pumpEff, nPumps=nPumps, speedLimFactor=speedLimFactor, pumpNominalRPM=pumpNominalRPM, pumpImpellerDiaFactor=pumpImpellerDiaFactor, iniT=initialT, iniP=initialP, refT=refT, refP=refP, refDensity=refDensity}
      mask prompts: extFluidMdot "External liquid loop mass flow rate vector (kg/s)"; extFluidPrDrop "External liquid loop pressure drop vector (kPa)"; extFluidVol "External liquid volume in heat exchanger (m^3)"; extFluidPipeArea "External liquid loop pipe cross-sectional area (m^2)"; intFluidMdot "Internal liquid loop mass flow rate vector (kg/s)"; intFluidPrDrop "Internal liquid loop pressure drop vector (kPa)"; intFluidVol "Internal liquid volume in heat exchanger (m^3)"; intFluidPipeArea "Internal liquid loop pipe cross-sectional area (m^2)"; spDissipationTbl "Specific dissipation table, SD[mdot_int,mdot_ext] (kW/K)"; effPipeLen "Effective pipe length for rack cooling (m)"; pumpCapacityVec "Reference capacity vector for each pump (m^3/s)"; pumpRefHeadVec "Reference head vector for each pump (m)"; pumpRefBrkPowVec "Reference brake power vector (kW)"; pumpEff "Electrical efficiency vector, 0-1 (-)"; nPumps "Total number of pumps (-)"; speedLimFactor "Pump speed upper limit factor (-)"; pumpNominalRPM "Pump nominal rating (rpm)"; pumpImpellerDiaFactor "Impeller diameter scale factor (-)"; iniT "Initial temperature (K)"; iniP "Initial pressure (MPa)"; refT "Reference flow temperature (K)"; refP "Reference flow pressure (MPa)"; refDensity "Reference density for internal liquid (kg/m^3)"
      settings: CopyFcn=set_param(gcbh,'LinkStatus','none');  PortSchema="{\"entries\":[{\"content\":{\"sides\":[{\"content\":{\"connectorIds\":[\"LConn1\",\"LConn2\",\"LConn3\"]},\"type\":\"ConnectorPlacement.EquallySpacedRectSide\",\"uuid\":\"dd9276e8-a048-49df-a05c-f18b45aafce3\"},{\"content\":{\"connectorIds\":[\"RConn1\",\"RConn2\"],\"side\":\"RIGHT\"},\"type\":\"ConnectorPlacement.EquallySpacedRectSide\",\"uuid\":\"f4cbe01b-cfd4-4d60-aff7-a07955033ed5\"},{\"content\":{\"connectorIds\":[\"LConn4\"],\"side\":\"TOP\"},\"type\":\"ConnectorPlacement.EquallySpacedRectSide\",\"uuid\":\"ad27df56-4241-452c-8570-6a66062dd2f2\"}]},\"type\":\"ConnectorPlacement.EquallySpacedConnector\",\"uuid\":\"0333b5f9-1896-45e0-922d-790b0e5dd980\"}],\"packageUris\":[\"http://schema.mathworks.com/mf0/Connector/R2020b\"],\"version\":\"1.0\"}"
      mask Help: web("DocumentationCDUTL.html")
      mask DialogControl Container5 Prompt: Heat Exchanger
      mask DialogControl Container8 Prompt: Set External Fluid Properties
      mask DialogControl Container7 Prompt: Set Internal Fluid Properties
      mask DialogControl Container9 Prompt: Heat Transfer
      mask DialogControl Container6 Prompt: Pumps
      mask DialogControl Container4 Prompt: Initial Conditions
      mask Display: image('icon_CDUthermalLiquid.png');
  Flow Multiplier : datacenter_lib/Flow Multiplier
      settings: InternalSimscapePortConfiguration="{\"Bottom\":[],\"Left\":[{\"id\":\"A\",\"label\":\"A\",\"type\":\"foundation.thermal_liquid.thermal_liquid\"}],\"Right\":[{\"id\":\"B\",\"label\":\"B\",\"type\":\"foundation.thermal_liquid.thermal_liquid\"}],\"Top\":[{\"id\":\"Na\",\"label\":\"Na\",\"type\":\"input\"},{\"id\":\"Nb\",\"label\":\"Nb\",\"type\":\"input\"}]}"
  Flow Multiplier1 : datacenter_lib/Flow Multiplier
      settings: InternalSimscapePortConfiguration="{\"Bottom\":[],\"Left\":[{\"id\":\"A\",\"label\":\"A\",\"type\":\"foundation.thermal_liquid.thermal_liquid\"}],\"Right\":[{\"id\":\"B\",\"label\":\"B\",\"type\":\"foundation.thermal_liquid.thermal_liquid\"}],\"Top\":[{\"id\":\"Na\",\"label\":\"Na\",\"type\":\"input\"},{\"id\":\"Nb\",\"label\":\"Nb\",\"type\":\"input\"}]}"
  One : fl_lib/Physical Signals/Sources/PS Constant  constant=1
  PDU Racks : Subsystem  mask{nTrays=nTrays, nRacks=nRacks, trayMass=trayMass, trayCp=trayCp, trayThermalR=trayThermalR, nGPU=nGPU, gpuTDPperDie=gpuTDPperDie, gpuIdlePower=gpuIdlePower, gpuHBMpower=gpuHBMpower, gpuExponent=gpuExponent, gpuHBMutil=gpuHBMutil, gpuLeakage=gpuLeakage, gpuNominalDieT=gpuNominalDieT, gpuDieThermalC=gpuDieThermalC, gpuHeatSinkR=gpuHeatSinkR, gpuSurfArea=gpuSurfArea, gpuAmbientR=gpuAmbientR, nCPU=nCPU, cpuTDPperSocket=cpuTDPperSocket, cpuIdlePower=cpuIdlePower, cpuExponent=cpuExponent, cpuLeakage=cpuLeakage, cpuNominalDieT=cpuNominalDieT, cpuDieThermalC=cpuDieThermalC, cpuHeatSinkR=cpuHeatSinkR, cpuSurfArea=cpuSurfArea, cpuAmbientR=cpuAmbientR, initialT=initialT, htc=htc}
      mask prompts: nTrays "Number of IT trays per rack (-)"; nRacks "Number of racks (-)"; trayMass "Tray mass (kg)"; trayCp "Tray specific heat capacity (J/kg*K)"; trayThermalR "Tray to external thermal resistance (K/W)"; nGPU "Number of GPU per tray (-)"; gpuTDPperDie "GPU TDP per die (W)"; gpuIdlePower "GPU idle power (W)"; gpuHBMpower "HBM power per GPU (W)"; gpuExponent "GPU power utilization exponent (-)"; gpuHBMutil "HBM utilization as fraction of compute utilization (-)"; gpuLeakage "Leakage increase per K above nominal temperature (W/K)"; gpuNominalDieT "Nominal die temperature at TDP (K)"; gpuDieThermalC "GPU die thermal capacitance (J/K)"; gpuHeatSinkR "GPU die-heat-sink thermal resistance (K/W)"; gpuSurfArea "Surface area per die for ambient heat transfer (m^2)"; gpuAmbientR "GPU die-ambient thermal resistance (K/W)"; nCPU "Number of CPU per tray (-)"; cpuTDPperSocket "CPU TDP per socket (W)"; cpuIdlePower "CPU idle power per socket (W)"; cpuExponent "CPU power utilization exponent (-)"; cpuLeakage "Leakage increase per K above nominal temperature (W/K)"; cpuNominalDieT "Nominal die temperature at TDP (K)"; cpuDieThermalC "CPU die thermal capacitance (J/K)"; cpuHeatSinkR "CPU die-heat-sink thermal resistance (K/W)"; cpuSurfArea "Surface area per die for ambient heat transfer (m^2)"; cpuAmbientR "CPU die-ambient thermal resistance (K/W)"; initialT "Initial temperature (K)"; htc "Heat transfer coefficient to ambient (W/m^2.K)"
      settings: CopyFcn=set_param(gcbh,'LinkStatus','none');  PortSchema="{\"entries\":[{\"content\":{\"sides\":[{\"content\":{\"connectorIds\":[\"LConn1\",\"LConn2\",\"LConn3\"]},\"type\":\"ConnectorPlacement.EquallySpacedRectSide\",\"uuid\":\"1a9a884a-dab1-4495-bf62-c6b2de6c1039\"},{\"content\":{\"connectorIds\":[\"RConn1\",\"RConn2\",\"RConn3\"],\"side\":\"RIGHT\"},\"type\":\"ConnectorPlacement.EquallySpacedRectSide\",\"uuid\":\"05c53434-51c1-4fee-b885-c321dcda8b6b\"},{\"content\":{\"side\":\"TOP\"},\"type\":\"ConnectorPlacement.EquallySpacedRectSide\",\"uuid\":\"c7b5c534-d596-4858-a133-27f005e6c9d4\"},{\"content\":{\"connectorIds\":[\"RConn4\"],\"side\":\"BOTTOM\"},\"type\":\"ConnectorPlacement.EquallySpacedRectSide\",\"uuid\":\"693f3c99-4296-4d86-bfcc-da753d3e576f\"}]},\"type\":\"ConnectorPlacement.EquallySpacedConnector\",\"uuid\":\"ed91c467-c4d0-403f-af16-bac0257594fd\"}],\"packageUris\":[\"http://schema.mathworks.com/mf0/Connector/R2020b\"],\"version\":\"1.0\"}"
      mask Help: web("DocumentationPDURacks.html")
      mask DialogControl Container10 Prompt: PDU Racks
      mask DialogControl getRatingButton Prompt: Get Rating
      mask DialogControl Container9 Prompt: IT Tray
      mask DialogControl Container6 Prompt: GPU
      mask DialogControl Container7 Prompt: CPU
      mask DialogControl Container8 Prompt: Initial Conditions
      mask Display: image('icon_PDURacks.png');
  PS Product : fl_lib/Physical Signals/Functions/PS Product
  PS Product1 : fl_lib/Physical Signals/Functions/PS Product
  Thermal Multiplier : datacenter_lib/Thermal Multiplier
      settings: InternalSimscapePortConfiguration="{\"Bottom\":[],\"Left\":[{\"id\":\"A\",\"label\":\"A\",\"type\":\"foundation.thermal.thermal\"}],\"Right\":[{\"id\":\"B\",\"label\":\"B\",\"type\":\"foundation.thermal.thermal\"}],\"Top\":[{\"id\":\"Na\",\"label\":\"Na\",\"type\":\"input\"},{\"id\":\"Nb\",\"label\":\"Nb\",\"type\":\"input\"}]}"
  nAssemblies : fl_lib/Physical Signals/Sources/PS Constant  constant=nAssembly
  U_gpu : PMIOPort  Side=Left
  U_cpu : PMIOPort  Port=2  Side=Left
  S_cdu : PMIOPort  Port=3  Side=Left
  N_cdu : PMIOPort  Port=4  Side=Left
  Ha : PMIOPort  Port=5  Side=Left
  T_gpu : PMIOPort  Port=6  Side=Right
  T_cpu : PMIOPort  Port=7  Side=Right
  P_pdu : PMIOPort  Port=8  Side=Right
  P_cdu : PMIOPort  Port=9  Side=Right
  Ae : PMIOPort  Port=10  Side=Right
  Be : PMIOPort  Port=11  Side=Right
  connections:
  PDU Racks/RConn4 -- CDU (TL)/LConn4
  PDU Racks/RConn3 -- T_cpu/RConn1
  PDU Racks/LConn2 -- U_cpu/RConn1
  CDU (TL)/LConn2 -- N_cdu/RConn1
  PDU Racks/RConn2 -- T_gpu/RConn1
  PDU Racks/LConn1 -- U_gpu/RConn1
  CDU (TL)/LConn1 -- S_cdu/RConn1
  PDU Racks/LConn3 -- Thermal Multiplier/RConn1
  Ha/RConn1 -- Thermal Multiplier/LConn1
  Flow Multiplier/LConn1 -- Ae/RConn1
  Flow Multiplier/RConn1 -- CDU (TL)/LConn3
  Flow Multiplier1/RConn1 -- Be/RConn1
  Flow Multiplier1/LConn1 -- CDU (TL)/RConn2
  One/RConn1 -- Flow Multiplier/LConn2 -- Flow Multiplier1/LConn3 -- Thermal Multiplier/LConn2
  nAssemblies/RConn1 -- PS Product1/LConn1 -- Flow Multiplier1/LConn2 -- PS Product/LConn1 -- Thermal Multiplier/LConn3 -- Flow Multiplier/LConn3
  PS Product/LConn2 -- PDU Racks/RConn1
  PS Product/RConn1 -- P_pdu/RConn1
  PS Product1/LConn2 -- CDU (TL)/RConn1
  P_cdu/RConn1 -- PS Product1/RConn1
